simulink model "vco_2"  (Simulink 7.4)
settings: Solver=ode45  StartTime=0.0  StopTime=2e-4  RelTol=1e-5
StartFcn:
  | tic
StopFcn:
  | trun=toc
undefined symbols (not defined in the file or in its folder): Fs, sided, Two
libraries: powerlib x11, dsparch4 x2, simpower_extensions_1 x2, simulink x1, dspsnks4 x1
settings Model: Creator=dbenson  LastModifiedBy=Dick
settings DataIOCC: SignalLoggingName=sigsOut
settings OptimizationCC: InlineInvariantSignals=on  InitFltsAndDblsToZero=on
settings DebuggingCC: SaveWithParameterizedLinksMsg=none  SignalResolutionControl=TryResolveAllWithWarning  SolverPrmCheckMsg=none  MultiTaskDSMMsg=warning  MultiTaskCondExecSysMsg=none  StrictBusMsg=None
settings HardwareCC: TargetUnknown=on
settings RTWCC: IncludeERTFirstTime=on
settings GRTTargetCC: TargetFcnLib=ansi_tfl_tmw.mat

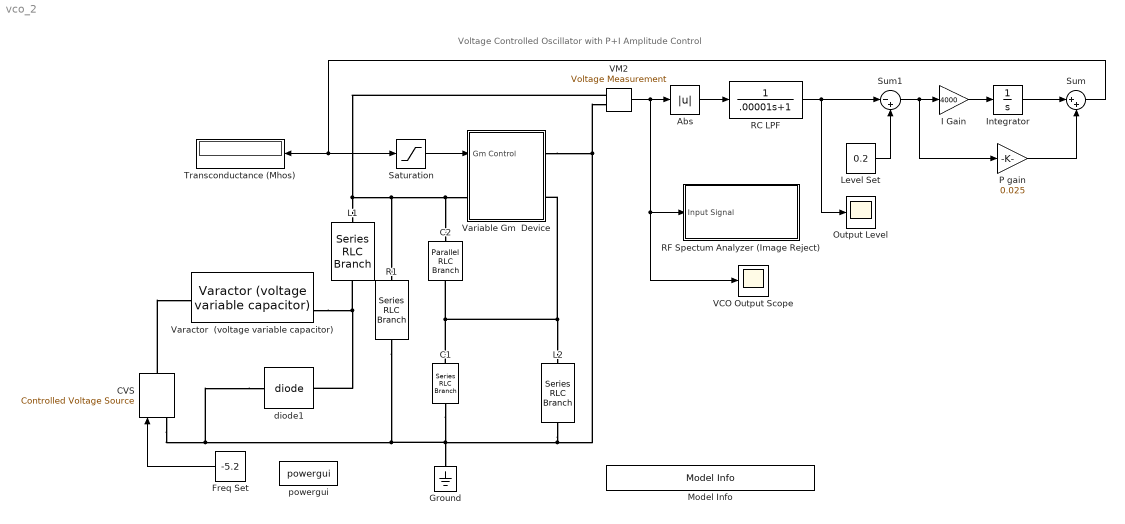
== system vco_2 ==
  note: Voltage Controlled Oscillator with P+I Amplitude Control
  Abs : Abs  SaturateOnIntegerOverflow=on
  C1 : powerlib/Elements/Series RLC Branch  DialogController=POWERSYS.PowerSysDialog  PhysicalDomain=powersysdomain  SubClassName=unknown  LeftPortType=p1  RightPortType=p1  LConnTagsString=__new0  RConnTagsString=__new0  BranchType=C  Resistance=1.0  Inductance=1.0  SetiL0=off  InitialCurrent=0  Capacitance=1500e-12  Setx0=off  InitialVoltage=0  Measurements=None
  C2 : powerlib/Elements/Parallel RLC Branch  DialogController=POWERSYS.PowerSysDialog  PhysicalDomain=powersysdomain  SubClassName=unknown  LeftPortType=p1  RightPortType=p1  LConnTagsString=a  RConnTagsString=__new0  BranchType=C  Resistance=1.0  Inductance=1.0  SetiL0=off  InitialCurrent=0  Capacitance=300e-12  Setx0=off  InitialVoltage=0  Measurements=None
  CVS : powerlib/Electrical Sources/Controlled Voltage Source  Description=source block  DialogController=POWERSYS.PowerSysDialog  SystemSampleTime=-1  Initialize=off  Source_Type=AC  Amplitude=0  Phase=0  Frequency=0  Measurements=None
      settings: AttributesFormatString=\n
  Freq Set : Constant  Value=-5.2  OutDataType=sfix(16)  OutScaling=2^0
  Ground : powerlib/Elements/Ground  DialogController=POWERSYS.PowerSysDialog  PhysicalDomain=powersysdomain  SubClassName=unknown  LeftPortType=p1  RightPortType=p1  LConnTagsString=a
  I Gain : Gain  Gain=4000  ParameterDataType=sfix(16)  ParameterScaling=2^0  OutDataType=sfix(16)  OutScaling=2^0  SaturateOnIntegerOverflow=on  OutDataTypeStr=Inherit: Same as input  ParamDataTypeStr=Inherit: Same as input
  Integrator : Integrator  InitialCondition=.025
  L1 : powerlib/Elements/Series RLC Branch  DialogController=POWERSYS.PowerSysDialog  PhysicalDomain=powersysdomain  SubClassName=unknown  LeftPortType=p1  RightPortType=p1  LConnTagsString=__new0  RConnTagsString=__new0  BranchType=RL  Resistance=1 % Inductor Loss  Inductance=3e-6  SetiL0=off  InitialCurrent=0  Capacitance=1.0  Setx0=off  InitialVoltage=0  Measurements=None
  L2 : powerlib/Elements/Series RLC Branch  DialogController=POWERSYS.PowerSysDialog  PhysicalDomain=powersysdomain  SubClassName=unknown  LeftPortType=p1  RightPortType=p1  LConnTagsString=__new0  RConnTagsString=__new0  BranchType=L  Resistance=1.0  Inductance=1e-3  SetiL0=off  InitialCurrent=0  Capacitance=1.0  Setx0=off  InitialVoltage=0  Measurements=None
  Level Set : Constant  Value=0.2  OutDataType=sfix(16)  OutScaling=2^0
  Model Info : simulink/Model-Wide Utilities/Model Info  SystemSampleTime=-1  InitialBlockCM=None  BlockCM=None  Frame=on  DisplayStringWithTags=Copywrite 2005-2010 The MathWorks, Inc.  HorizontalTextAlignment=Center  LeftAlignmentValue=0.5  SourceBlockDiagram=vco_2  TagMaxNumber=20
  Output Level : Scope
      settings: TimeRange=0.0006000000000000001  YMin=0.199925  YMax=0.200075  SaveName=ScopeData2  MaxDataPoints=50000  Decimation=100
  P gain : Gain  Gain=0.025  ParameterDataType=sfix(16)  ParameterScaling=2^0  OutDataType=sfix(16)  OutScaling=2^0  SaturateOnIntegerOverflow=on  OutDataTypeStr=Inherit: Same as input  ParamDataTypeStr=Inherit: Same as input
  R1 : powerlib/Elements/Series RLC Branch  DialogController=POWERSYS.PowerSysDialog  PhysicalDomain=powersysdomain  SubClassName=unknown  LeftPortType=p1  RightPortType=p1  LConnTagsString=__new0  RConnTagsString=__new0  BranchType=R  Resistance=10000  Inductance=1.0  SetiL0=off  InitialCurrent=0  Capacitance=1.0  Setx0=off  InitialVoltage=0  Measurements=None
  RC LPF : TransferFcn  Denominator=[.00001 1]
  RF Spectum Analyzer (Image Reject) : Subsystem  Description=Spectrum Analyzer  mask{BW=4e6, Fc=15.75e6, Zo=50}
      mask prompts: BW "Bandwidth"; Fc "Center Freq"; Zo "Load Resistance"
      mask Display: fprintf('Spectrum Analyzer \n Fc=%7.2f MHz \n BW=%7.2f MHz',Fc/1e6,BW/1e6)
  Saturation : Saturate  UpperLimit=0.1  LowerLimit=0
  Sum : Sum  Inputs=|++  OutDataType=sfix(16)  OutScaling=2^0  SaturateOnIntegerOverflow=on
  Sum1 : Sum  Inputs=|-+  OutDataType=sfix(16)  OutScaling=2^0  SaturateOnIntegerOverflow=on
  Transconductance (Mhos) : Display
  VCO Output Scope : Scope
      settings: TimeRange=2.5e-007  YMin=0.12  YMax=0.28  MaxDataPoints=50000
  VM2 : powerlib/Measurements/Voltage Measurement  Tag=PoWeRsYsTeMmEaSuReMeNt  DialogController=POWERSYS.PowerSysDialog  SystemSampleTime=-1  PhasorSimulation=off  OutputType=Magnitude  PSBequivalent=0
  Varactor  (voltage variable capacitor) : simpower_extensions_1/Varactor  (voltage variable capacitor)  SystemSampleTime=-1  Cjo=100e-12  Vj=0.7  M=0.5  Cp=5e-12
  Variable Gm  Device : Subsystem
  diode1 : simpower_extensions_1/diode  SystemSampleTime=-1  Is=1e-8  Rfwd=1
  powergui : powerlib/powergui  SystemSampleTime=-1  SimulationMode=Continuous  SampleTime=0  frequency=60  SPID=off  DisableSnubberDevices=off  DisableRonSwitches=off  DisableVfSwitches=off  SwTol=0  Interpol=off  frequencyindice=0  echomessages=off  HookPort=off  DisplayEquations=off  FunctionMessages=off  EnableUseOfTLC=off  x0status=blocks  RestoreLinks=warning  Frange=[0:2:500]  Ylog=off  Xlog=on  ShowGrid=off  save=off  variable=ZData  ZoomFFT=on  StartTime=0.0  cycles=1  DisplayStyle=1  fundamental=60  FreqAxis=off  MaxFrequency=1000  frequencyindicesteady=1  RmsSteady=1  display=off  Ts=0  methode=off
  wires:
  Freq Set/1 -> CVS/1
  Saturation/1 -> Variable Gm  Device/1(Gm Control)
  VM2/1 -> Abs/1, VCO Output Scope/1, RF Spectum Analyzer (Image Reject)/1(Input Signal)
  Abs/1 -> RC LPF/1
  RC LPF/1 -> Output Level/1, Sum1/1
  Sum1/1 -> I Gain/1, P gain/1
  Level Set/1 -> Sum1/2
  I Gain/1 -> Integrator/1
  Integrator/1 -> Sum/1
  P gain/1 -> Sum/2
  Sum/1 -> Saturation/1, Transconductance (Mhos)/1
  connections:
  L2/LConn1 -- Variable Gm  Device/RConn2 -- C1/LConn1 -- C2/RConn1
  diode1/LConn1 -- CVS/LConn1 -- R1/RConn1 -- Variable Gm  Device/RConn1 -- VM2/LConn2 -- L2/RConn1 -- C1/RConn1 -- Ground/LConn1
  CVS/RConn1 -- Varactor  (voltage variable capacitor)/LConn1
  diode1/RConn1 -- Varactor  (voltage variable capacitor)/RConn1 -- L1/RConn1
  L1/LConn1 -- VM2/LConn1 -- Variable Gm  Device/LConn1 -- C2/LConn1 -- R1/LConn1

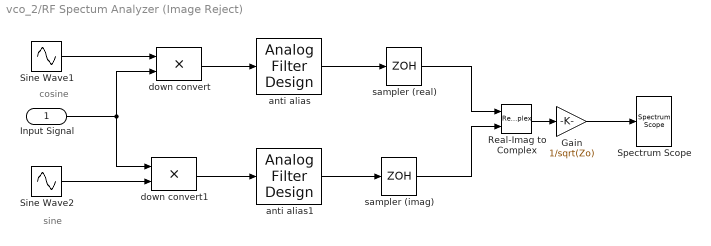
== system vco_2/RF Spectum Analyzer (Image Reject) ==
  note: cosine
  note: sine
  Input Signal : Inport  OutDataType=sfix(16)  OutScaling=2^0
  Gain : Gain  Gain=1/sqrt(Zo)  ParameterDataType=fixdt(1, 16)  ParameterScaling=2^0  OutDataType=fixdt(1, 16)  OutScaling=2^0
  Real-Imag to Complex : RealImagToComplex
  Sine Wave1 : Sin  Amplitude=sqrt(2)  Bias=0  Frequency=2*pi*(Fc)  Phase=-pi/2  Samples=10  SampleTime=0  Offset=0
  Sine Wave2 : Sin  Amplitude=sqrt(2)  Bias=0  Frequency=2*pi*(Fc)  Phase=0  Samples=10  SampleTime=0  Offset=0
  Spectrum Scope : dspsnks4/Spectrum Scope  DialogController=dspdialog.SpectrumScope  DialogControllerArgs=DataTag0  SystemSampleTime=-1  ScopeProperties=on  Domain=Frequency  HorizSpan=1  UseBuffer=on  BufferSize=256  Overlap=64  inpFftLenInherit=off  FFTlength=128  numAvg=2  DisplayProperties=off  AxisGrid=on  Memory=off  FrameNumber=on  AxisLegend=off  AxisZoom=off  OpenScopeAtSimStart=on  OpenScopeImmediately=off  FigPos=[626 37 392 254]  AxisProperties=off  XUnits=Hertz  XRange=Two-sided ((-Fs/2...Fs/2])  XDisplay=0  InheritXIncr=on  XIncr=1.0  XLabel=Samples  XLimit=Auto  YUnits=dBm  XMax=1  XMin=0  YLabel=dBm  LineProperties=off  wintypeSpecScope=Hann  RsSpecScope=50  betaSpecScope=5  winsampSpecScope=Periodic  XAxisParamsVer=6.9
      settings: YMin=-100  YMax=0
  anti alias : dsparch4/Analog Filter Design  method=Elliptic  filttype=Lowpass  N=9  Wlo=BW*pi  Whi=80  Rp=1.2  Rs=100
  anti alias1 : dsparch4/Analog Filter Design  method=Elliptic  filttype=Lowpass  N=9  Wlo=BW*pi  Whi=80  Rp=1.2  Rs=100
  down convert : Product  OutDataType=sfix(16)  OutScaling=2^0  SaturateOnIntegerOverflow=on  InputSameDT=on  OutDataTypeStr=Inherit: Same as first input
  down convert1 : Product  OutDataType=sfix(16)  OutScaling=2^0  SaturateOnIntegerOverflow=on  InputSameDT=on  OutDataTypeStr=Inherit: Same as first input
  sampler (imag) : ZeroOrderHold  SampleTime=1/(1.28*BW)
  sampler (real) : ZeroOrderHold  SampleTime=1/(1.28*BW)
  wires:
  Input Signal/1 -> down convert/2, down convert1/1
  down convert/1 -> anti alias/1
  anti alias/1 -> sampler (real)/1
  Sine Wave1/1 -> down convert/1
  Sine Wave2/1 -> down convert1/2
  anti alias1/1 -> sampler (imag)/1
  down convert1/1 -> anti alias1/1
  sampler (real)/1 -> Real-Imag to Complex/1
  sampler (imag)/1 -> Real-Imag to Complex/2
  Real-Imag to Complex/1 -> Gain/1
  Gain/1 -> Spectrum Scope/1

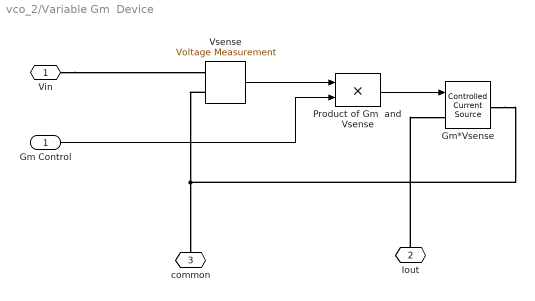
== system vco_2/Variable Gm  Device ==
  Gm Control : Inport  OutDataType=sfix(16)  OutScaling=2^0
  Gm*Vsense : powerlib/Electrical Sources/Controlled Current Source  Description=source block  DialogController=POWERSYS.PowerSysDialog  SystemSampleTime=-1  Initialize=off  Source_Type=AC  Amplitude=-0.025  Phase=0  Frequency=0  Measurements=None
      settings: AttributesFormatString=\n
  Product of Gm  and  Vsense : Product  OutDataType=sfix(16)  OutScaling=2^0  SaturateOnIntegerOverflow=on  OutDataTypeStr=Inherit: Same as first input
  Vsense : powerlib/Measurements/Voltage Measurement  Tag=PoWeRsYsTeMmEaSuReMeNt  DialogController=POWERSYS.PowerSysDialog  SystemSampleTime=-1  PhasorSimulation=off  OutputType=Magnitude  PSBequivalent=0
  Vin : PMIOPort  Port=1  Side=Left
  Iout : PMIOPort  Port=2  Side=Right
  common : PMIOPort  Port=3  Side=Right
  wires:
  Vsense/1 -> Product of Gm  and  Vsense/1
  Product of Gm  and  Vsense/1 -> Gm*Vsense/1
  Gm Control/1 -> Product of Gm  and  Vsense/2
  connections:
  Vsense/LConn2 -- common/RConn1 -- Gm*Vsense/RConn1
  Vin/RConn1 -- Vsense/LConn1
  Iout/RConn1 -- Gm*Vsense/LConn1
